simulink model "Acc_Dec_Check"  (R2020a)
settings: Solver=FixedStepAuto  StartTime=0.0  StopTime=10.0  RelTol=1e-3
libraries: simulink x3
settings Model: OrderedModelArguments=off  Creator=ashok  LastModifiedBy=ashok

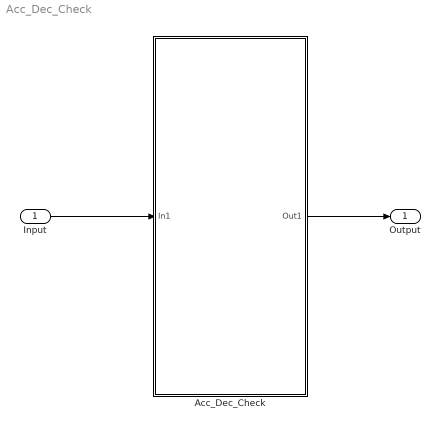
== system Acc_Dec_Check ==
  Input : Inport
  Acc_Dec_Check : Subsystem
  Output : Outport
  wires:
  Input/1 -> Acc_Dec_Check/1(In1)
  Acc_Dec_Check/1(Out1) -> Output/1

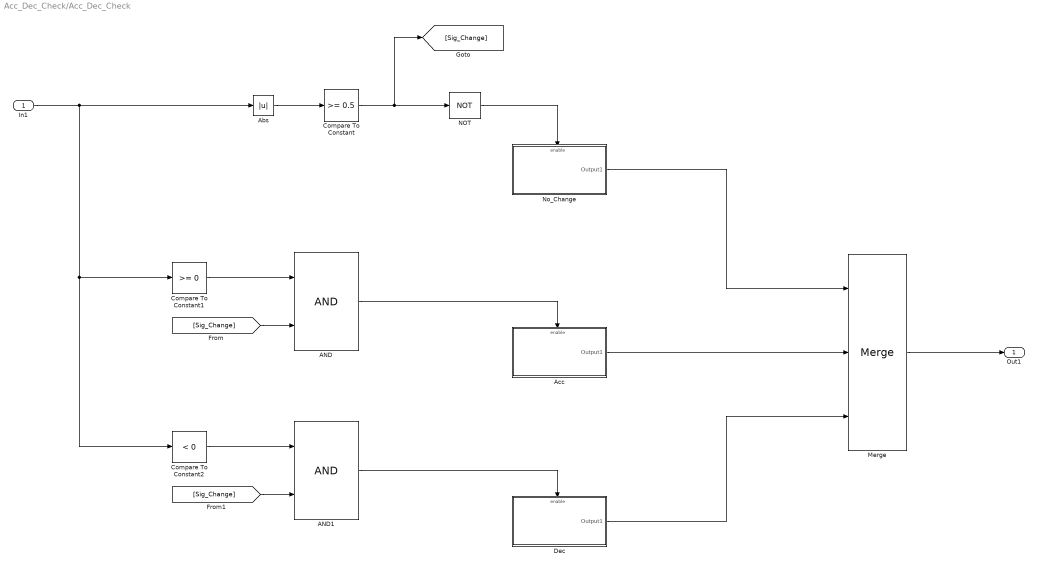
== system Acc_Dec_Check/Acc_Dec_Check ==
  In1 : Inport
  AND : Logic  AllPortsSameDT=off  OutDataTypeStr=boolean
  AND1 : Logic  AllPortsSameDT=off  OutDataTypeStr=boolean
  Abs : Abs
  Acc : Subsystem
  Compare To Constant : simulink/Logic and Bit Operations/Compare To Constant  relop=>=  const=0.5  OutDataTypeStr=boolean
  Compare To Constant1 : simulink/Logic and Bit Operations/Compare To Constant  relop=>=  const=0  OutDataTypeStr=boolean
  Compare To Constant2 : simulink/Logic and Bit Operations/Compare To Constant  relop=<  const=0  OutDataTypeStr=boolean
  Dec : Subsystem
  Merge : Merge  Inputs=3
  NOT : Logic  Operator=NOT  AllPortsSameDT=off  OutDataTypeStr=boolean
  No_Change : Subsystem
  Out1 : Outport
  wires:
  Compare To Constant2/1 -> AND1/1
  Compare To Constant1/1 -> AND/1
  [Sig_Change] -> AND1/2
  NOT/1 -> No_Change/Enable
  [Sig_Change] -> AND/2
  Dec/1(Output1) -> Merge/3
  No_Change/1(Output1) -> Merge/1
  Acc/1(Output1) -> Merge/2
  Merge/1 -> Out1/1
  Compare To Constant/1 -> [Sig_Change], NOT/1
  Abs/1 -> Compare To Constant/1
  AND/1 -> Acc/Enable
  In1/1 -> Compare To Constant1/1, Compare To Constant2/1, Abs/1
  AND1/1 -> Dec/Enable

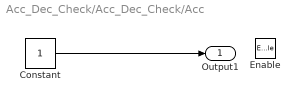
== system Acc_Dec_Check/Acc_Dec_Check/Acc ==
  Enable : EnablePort
  Constant : Constant
  Output1 : Outport
  wires:
  Constant/1 -> Output1/1

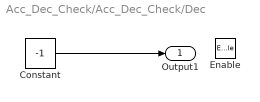
== system Acc_Dec_Check/Acc_Dec_Check/Dec ==
  Enable : EnablePort
  Constant : Constant  Value=-1
  Output1 : Outport
  wires:
  Constant/1 -> Output1/1

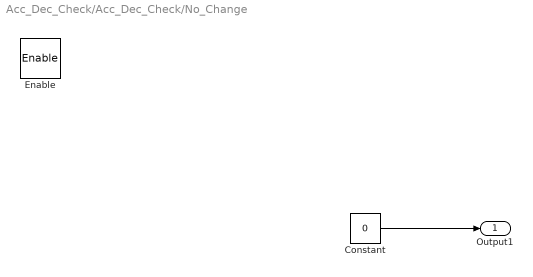
== system Acc_Dec_Check/Acc_Dec_Check/No_Change ==
  Enable : EnablePort
  Constant : Constant  Value=0
  Output1 : Outport
  wires:
  Constant/1 -> Output1/1
